simulink model "movement"  (R2021b)
settings: Solver=VariableStepAuto  StartTime=0.0  StopTime=10.0  RelTol=1e-3
libraries: arduinolib x4
settings Model: Creator=Aazam  LastModifiedBy=Aazam

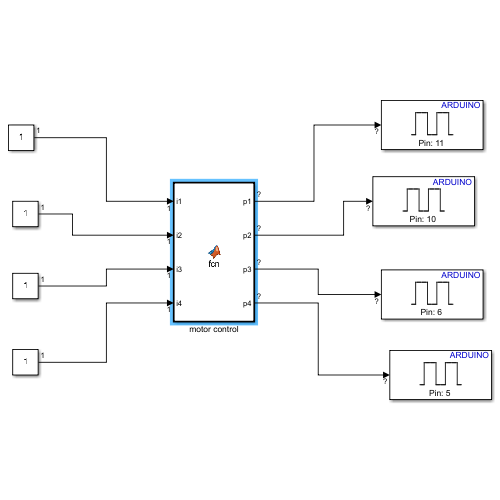
[thumbnail: Simulink's stored preview of the top-level diagram]
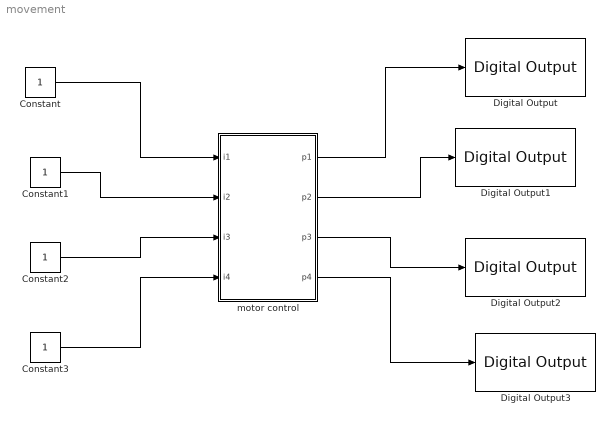
== system movement ==
  Constant{,1..3} (4 alike) : Constant
  Digital Output : arduinolib/Digital Output  pinNumber=11  Direction=output  blockPlatform=arduino
  Digital Output1 : arduinolib/Digital Output  pinNumber=10  Direction=output  blockPlatform=arduino
  Digital Output2 : arduinolib/Digital Output  pinNumber=6  Direction=output  blockPlatform=arduino
  Digital Output3 : arduinolib/Digital Output  pinNumber=5  Direction=output  blockPlatform=arduino
  motor control : MATLAB Function  TreatAsAtomicUnit=on
  wires:
  Constant/1 -> motor control/1(i1)
  Constant1/1 -> motor control/2(i2)
  Constant2/1 -> motor control/3(i3)
  Constant3/1 -> motor control/4(i4)
  motor control/1(p1) -> Digital Output/1
  motor control/2(p2) -> Digital Output1/1
  motor control/3(p3) -> Digital Output2/1
  motor control/4(p4) -> Digital Output3/1

== matlab function movement/motor control ==
  data: i1 input; p1 output; i2 input; i3 input; i4 input; p2 output; p3 output; p4 output
function [p1, p2, p3, p4] = fcn(i1, i2, i3, i4)
